simulink model "STEP1_demo1"  (Simulink 8.4)
settings: Solver=ode45  SolverMode=SingleTasking  StartTime=0.0  StopTime=inf  FixedStep=2/64e5  RelTol=1e-3
libraries: dspvision x2, dspsnks4 x1
settings Model: Creator=Schoenen  LastModifiedBy=Schoenen
settings DataIOCC: SignalLoggingName=sigsOut
settings OptimizationCC: ExpressionDepthLimit=128
settings DebuggingCC: SaveWithParameterizedLinksMsg=none  SignalResolutionControl=TryResolveAllWithWarning  SolverPrmCheckMsg=none  MultiTaskDSMMsg=warning  MultiTaskCondExecSysMsg=none  FcnCallInpInsideContextMsg=EnableAllAsError  StateNameClashWarn=none
settings HardwareCC: TargetUnknown=on
settings RTWCC: IncludeERTFirstTime=on

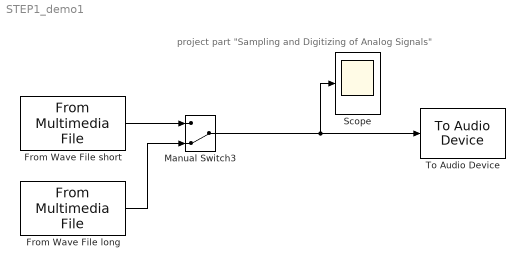
== system STEP1_demo1 ==
  note: project part "Sampling and Digitizing of Analog Signals"
  From Wave File long : dspvision/From Multimedia File  inputFilename=audio_sampled_with_8kHz.wav  loop=on  numPlays=1  outputStreams=Audio only  videoDataType=single  audioDataType=double  inheritSampleTime=on  userDefinedSampleTime=1/30  noAudioOutput=off  isIntensityVideo=off  fourcc=RGB  colorVideoFormat=Separate color signals  outputEOF=off  dataOrg=Column-major  audioFrameSize=1  computeAudioFrameSize=off  outSamplingMode=Sample based
  From Wave File short : dspvision/From Multimedia File  inputFilename=audio_in_8kHz.wav  loop=on  numPlays=1  outputStreams=Audio only  videoDataType=single  audioDataType=double  inheritSampleTime=on  userDefinedSampleTime=1/30  noAudioOutput=off  isIntensityVideo=off  fourcc=RGB  colorVideoFormat=Separate color signals  outputEOF=off  dataOrg=Column-major  audioFrameSize=1  computeAudioFrameSize=off  outSamplingMode=Sample based
  Manual Switch3 : ManualSwitch  CurrentSetting=0
  Scope : Scope
      settings: TimeRange=1  YMin=-1  YMax=1
  To Audio Device : dspsnks4/To Audio Device  deviceName=Default  inheritSampleRate=off  sampleRate=8000  deviceDatatype=Determine from input data type  autoBufferSize=on  bufferSize=4096  queueDuration=0.2  defaultOutputChannelMapping=on  outputChannelMapping=1:2  outputNumUnderrunSamples=off
  wires:
  From Wave File short/1 -> Manual Switch3/1
  From Wave File long/1 -> Manual Switch3/2
  Manual Switch3/1 -> To Audio Device/1, Scope/1
